simulink model "sf_mandelbrot_fixpt"  (R2017b)
settings: Solver=FixedStepDiscrete  StartTime=0.0  StopTime=inf  FixedStep=0.0005  RelTol=1e-3
CloseFcn:
  | sf_mandel_gui('close');
settings Model: FPTRunName=Active  ExtModeAutoUpdateStatusClock=off  Creator=The MathWorks, Inc.  LastModifiedBy=The MathWorks, Inc.
settings DataIOCC: LimitDataPoints=on  SaveFormat=Array  SaveOutput=off  SaveTime=off
settings OptimizationCC: BooleanDataType=off  ExpressionDepthLimit=2147483647  InitFltsAndDblsToZero=on  EfficientMapNaN2IntZero=off  LifeSpan=inf  BufferReusableBoundary=off
settings DebuggingCC: UnderspecifiedInitializationDetection=Classic  MergeDetectMultiDrivingBlocksExec=none  SignalResolutionControl=TryResolveAllWithWarning  MultiTaskDSMMsg=warning  MultiTaskCondExecSysMsg=none  IntegerOverflowMsg=none  FcnCallInpInsideContextMsg=warning  BusObjectLabelMismatch=none  StateNameClashWarn=warning  StrictBusMsg=None  SFUnexpectedBacktrackingDiag=warning  SFNoUnconditionalDefaultTransitionDiag=warning  SFExecutionAtInitializationDiag=none  IntegerSaturationMsg=none
settings HardwareCC: ProdBitPerPointer=32  ProdBitPerSizeT=32  ProdBitPerPtrDiffT=32  ProdLargestAtomicFloat=None  ProdIntDivRoundTo=Undefined  ProdEndianess=Unspecified  ProdWordSize=32  ProdHWDeviceType=32-bit Generic  TargetUnknown=on
settings ModelReferenceCC: PropagateSignalLabelsOutOfModel=off
settings SFSimCC: SFSimEcho=off  SimParseCustomCode=off
settings CodeAppCC: StateflowObjectComments=on
settings GRTTargetCC: TargetFcnLib=ansi_tfl_tmw.mat  TargetLangStandard=C89/C90 (ANSI)  GeneratePreprocessorConditionals=Disable all  CombineOutputUpdateFcns=off  GRTInterface=on
settings ConfigComp: CovMetricSettings=dcmtr  CovHtmlReporting=on  CovSaveCumulativeToWorkspaceVar=on  CovSaveSingleToWorkspaceVar=on  CovExternalEMLEnable=off  CovSFcnEnable=off

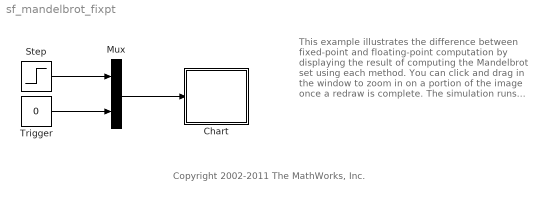
== system sf_mandelbrot_fixpt ==
  note: This example illustrates the difference between
      | fixed-point and floating-point computation by
      | displaying the result of computing the
      | Mandelbrot set using each method.
      |
      | You can click and drag in the window to zoom
      | in on a portion of the image once a redraw is
      | complete. The simulation runs until stopped.
  note: Copyright 2002-2011 The MathWorks, Inc.
  Chart : Stateflow chart  TreatAsAtomicUnit=on
  Mux : Mux  Inputs=2
  Step : Step  Time=0.1  SampleTime=0  ZeroCross=off
  Trigger : Constant  Value=0
  wires:
  Trigger/1 -> Mux/2
  Step/1 -> Mux/1
  Mux/1 -> Chart/Trigger

== stateflow chart sf_mandelbrot_fixpt/Chart ==
  state ii = mandel_double(a0,b0) [function]
    (default) -> (junction 43) : { ii = 0;
        |  r2 = 0;
        |  local_colors = colors; }
    (junction 41) -> (junction 43)
    (junction 44) -> (junction 41) : {
        | ii++;
        | }
    (junction 43) -> (junction 42) : {
        | bn = 2 * an * bn + b0;
        | an = r2 + a0;
        | r2 = an * an - bn * bn;
        | }
    (junction 42) -> (junction 40) [order 2]
    (junction 42) -> (junction 44) [order 1] : [ r2 < 4 && ii < local_colors ]
  state ii = mandel_fix(a0,b0) [function]
    (default) -> (junction 28) : { ii = 0;
        |  r2 = 0;
        |  local_colors = colors; }
    (junction 30) -> (junction 28)
    (junction 33) -> (junction 30) : {
        | ii++;
        | }
    (junction 28) -> (junction 29) : {
        | bn = 2 * an * bn + b0;
        | an = r2 + a0;
        | r2 = an * an - bn * bn;
        | }
    (junction 29) -> (junction 31) [order 2]
    (junction 29) -> (junction 33) [order 1] : [ r2 < 4 && ii < local_colors ]
  state Wait
    entry:ml.sf_mandel_gui("enter_wait");
  (default) -> (junction 36) : {
      | ml.sf_mandel_gui();
      | }
  Wait -> (junction 36) : Redraw
  (junction 36) -> (junction 45) : {
      | ml.sf_mandel_gui("exit_wait");
      | colors = ml.sf_mandel_gui("colors");
      |
      | pix_w = ml.sf_mandel_gui("pixel width");
      | pix_h  = ml.sf_mandel_gui("pixel height");
      |
      | real_left = ml.sf_mandel_gui("real left");
      | real_top = ml.sf_mandel_gui("real top");
      | real_w   = ml.sf_mandel_gui("real width");
      | real_h   = ml.sf_mandel_gui("real height");
      |
      | deltax = real_w / pix_w;
      | deltay = real_h / pix_h;
      |
      | i=1;
      | y0 = real_top;
      | ml.tic();
      | }
  (junction 37) -> Wait [order 2] : { ml.toc() }
  (junction 37) -> (junction 38) [order 1] : [ i <= pix_h ]
  (junction 45) -> (junction 37)
  (junction 35) -> (junction 37) [order 2] : {
      | ml.sf_mandel_gui(i,dbl_line,fix_line);
      | ml.sf_mandel_gui("update");
      | i++;
      | y0 -= deltay;
      | }
  (junction 38) -> (junction 39) : {
      | j = 1;
      | x = real_left;
      | }
  (junction 35) -> (junction 39) [order 1] : [ j <= pix_w]
  (junction 34) -> (junction 35) : {
      | j++;
      | x += deltax;
      | }
  (junction 39) -> (junction 32) : {
      | fix_line[j]  = mandel_fix(x,y0);
      | dbl_line[j] = mandel_double(x,y0);
      | }
  (junction 32) -> (junction 34)
  data: a0 function_input double; b0 function_input double; an temporary double; bn temporary double; ii function_output int32; local_colors temporary int32; r2 temporary double; a0 function_input fixdt(1,16,13); b0 function_input fixdt(1,16,13); an temporary fixdt(1,16,13); bn temporary fixdt(1,16,13); ii function_output int32; r2 temporary fixdt(1,32,26); local_colors temporary int32; real_left local double; real_w local double; pix_w local double; deltax local double; deltay local double; i local int32; y0 local double; j local int32; x local double; real_top local double; real_h local double; pix_h local double; colors local double; fix_line local double size=1024; dbl_line local double size=1024
  events: Start input EITHER_EDGE_EVENT; Redraw input EITHER_EDGE_EVENT
